simulink model "SEA_system_MPC_PID"  (R2023b)
settings: Solver=VariableStepAuto  StartTime=0.0  StopTime=10  FixedStep=0.005  RelTol=1e-3
values from neighbouring files (symbols this model uses):
  c1 = 0.6    [SEA_system.m]
  c2 = 0.6    [SEA_system.m]
  CoM1 = 0.117    [SEA_system.m]
  CoM2 = 0.045    [SEA_system.m]
  g = 9.81    [SEA_system.m]
  J1 = m1*L1^2/12 + m1*CoM1^2    (= 0.00579610927083)    [SEA_system.m]
  J2 = m2*L2^2/12 + m2*CoM2^2 + (mEE*(L2-CoM2)^2)    (= 0.00129963166667)    [SEA_system.m]
  k1 = 5.9*10^3    (= 5900)    [SEA_system.m]
  k2 = 5.9*10^3    (= 5900)    [SEA_system.m]
  L1 = 0.20075    [SEA_system.m]
  m1 = 0.340    (= 0.34)    [SEA_system.m]
  m2 = 0.140    (= 0.14)    [SEA_system.m]
  N1 = m1*CoM1^2 + J1 + m2*L1^2 + m2*CoM2^2 + J2    (= 0.0176755796875)    [SEA_system.m]
  N2 = m2*L1*CoM2    (= 0.001264725)    [SEA_system.m]
  N3 = m2*CoM2^2 + J2    (= 0.00158313166667)    [SEA_system.m]
libraries: simulink_extras x4, slpidlib x2, mpclib x1
settings Model: Creator=Master  LastModifiedBy=tpdnr
settings SolverCC: ZeroCrossAlgorithm=Adaptive
settings DebuggingCC: MaskedZcDiagnostic=none  IgnoredZcDiagnostic=none

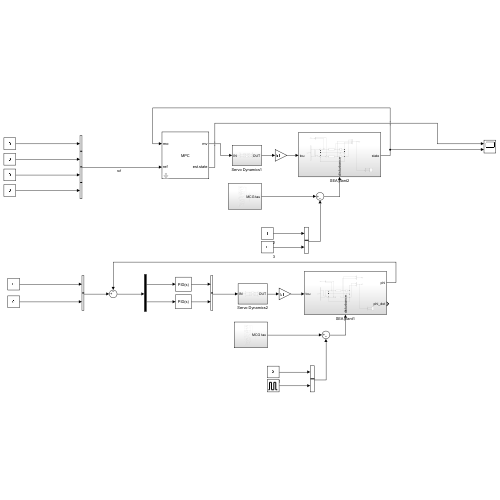
[thumbnail: Simulink's stored preview of the top-level diagram]
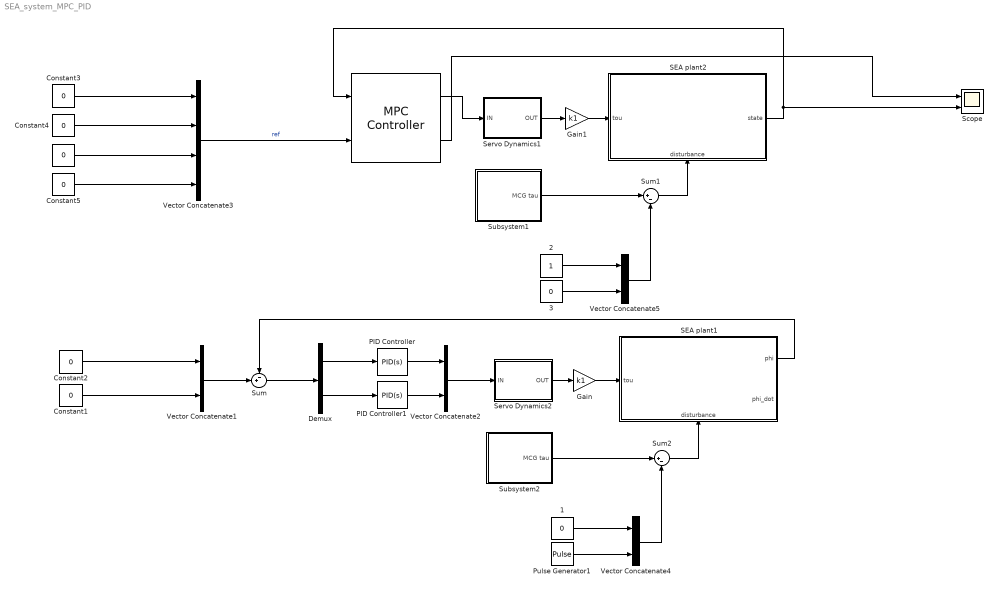
== system SEA_system_MPC_PID ==
  " " : Constant  Value=0
  "  " : mpclib/MPC Controller  SCDEnableBlockLinearizationSpecification=on  mpcobj=mpcobj  is_multiple=0  enable_value=0  return_u0=off  updateMPCinCallerWorkspace=on  md_inport=off  mv_inport=off  uref_inport=off  return_cost=off  return_mvseq=off  return_qpstatus=off  return_xseq=off  return_state=on  return_ovseq=off  state_inport=off  umin_inport=off  umax_inport=off  ymin_inport=off  ymax_inport=off  cc_inport=off  ywt_inport=off  uwt_inport=off  duwt_inport=off  rhoeps_inport=off  pm_inport=off  MaximumP=10  HorizonChoice=FixedHorizon  n_ts=0.01  n_p=10  n_mv=2  n_md=0  n_ud=0  n_mo=4  n_uo=0  BlockDataType=double  SampleTimeInherited=off  switch_inport=off
  "            1" : Constant  Value=0
  "            2" : Constant
  "            3" : Constant  Value=0
  Constant{1..5} (5 alike) : Constant  Value=0
  Demux : Demux  Outputs=2
  Gain : Gain  Gain=k1
  Gain1 : Gain  Gain=k1
  PID Controller : slpidlib/PID Controller  Controller=PID  Form=Parallel  TimeDomain=Continuous-time  UseExternalTs=off  SampleTime=-1  IntegratorMethod=Forward Euler  FilterMethod=Forward Euler  ControllerParametersSource=internal  P=5  I=1  UseKiTs=off  D=0  N=100  UseFilter=on  TunerSelectOption=Transfer Function Based (PID Tuner App)  InitialConditionSource=internal  InitialConditionForIntegrator=0  InitialConditionForFilter=0  DifferentiatorICPrevScaledInput=0  ExternalReset=none  TrackingMode=off  Kt=1  LimitOutput=off  SatLimitsSource=internal  UpperSaturationLimit=inf  LowerSaturationLimit=-inf  LinearizeAsGain=on  AntiWindupMode=none  Kb=1  LimitIntegrator=off  UpperIntegratorSaturationLimit=inf  LowerIntegratorSaturationLimit=-inf  POutMin=[]  POutMax=[]  IOutMin=[]  IOutMax=[]  DOutMin=[]  DOutMax=[]  NOutMin=[]  NOutMax=[]  SumOutMin=[]  SumOutMax=[]  SaturationOutMin=[]  SaturationOutMax=[]  PParamMin=[]  PParamMax=[]  IParamMin=[]  IParamMax=[]  DParamMin=[]  DParamMax=[]  NParamMin=[]  NParamMax=[]  KbParamMin=[]  KbParamMax=[]  KtParamMin=[]  KtParamMax=[]  KbOutMin=[]  KbOutMax=[]  KtOutMin=[]  KtOutMax=[]  IntegratorOutMin=[]  IntegratorOutMax=[]  FilterOutMin=[]  FilterOutMax=[]  SumI1OutMin=[]  SumI1OutMax=[]  SumI2OutMin=[]  SumI2OutMax=[]  SumI3OutMin=[]  SumI3OutMax=[]  SumI4OutMin=[]  SumI4OutMax=[]  SumDOutMin=[]  SumDOutMax=[]  DifferentiatorOutMin=[]  DifferentiatorOutMax=[]  FilterDiffOutCoefMin=[]  FilterDiffOutCoefMax=[]  ReciprocalOutMin=[]  ReciprocalOutMax=[]  SumDenOutMin=[]  SumDenOutMax=[]  SumNumOutMin=[]  SumNumOutMax=[]  DivideOutMin=[]  DivideOutMax=[]  UdiffTsProdOutMin=[]  UdiffTsProdOutMax=[]  NTsProdOutMin=[]  NTsProdOutMax=[]  UintegralTsProdOutMin=[]  UintegralTsProdOutMax=[]  UngainTsProdOutMin=[]  UngainTsProdOutMax=[]  ClampingZeroOutDataTypeStr=Inherit: Inherit via back propagation  ClampingZeroOutMin=[]  ClampingZeroOutMax=[]  FilterDenConstantOutDataTypeStr=Inherit: Inherit via back propagation  FilterDenConstantOutMin=[]  FilterDenConstantOutMax=[]  PCopyOutDataTypeStr=Inherit: Inherit via back propagation  PCopyOutMin=[]  PCopyOutMax=[]  NCopyOutDataTypeStr=Inherit: Inherit via back propagation  NCopyOutMin=[]  NCopyOutMax=[]  IntegratorContinuousStateAttributes=''  IntegratorStateMustResolveToSignalObject=off  IntegratorRTWStateStorageClass=Auto  FilterContinuousStateAttributes=''  FilterStateMustResolveToSignalObject=off  FilterRTWStateStorageClass=Auto  ParallelPVariant=InternalParameters  IdealPVariant=Disabled  IVariant=InternalParameters  DVariant=InternalParameters  IntegratorVariant=Continuous  SatVariant=Disabled  AWVariant=Passthrough  PCopyVariant=Disabled  TRVariant=Disabled  FdbkBlocksVariant=Forward  IdealPFdbkVariant=Disabled  SatFdbkVariant=Disabled  DerivativeFilterVariant=ContFilter  NVariant=InternalParameters  NCopyVariant=Disabled  FilterICVariant=InternalICsFilter  IntegratorICVariant=InternalICs  ExternalResetVariant=Disabled  TRSumVariant=Passthrough  SumFdbkVariant=Disabled  SumVariant=Sum_PID  TsampFilterVariant=InternalTs  TsampNgainVariant=Passthrough  TsampIntegralVariant=Disabled_SignalSpec  ExternalSaturationOutDataTypeStr=Inherit: Same as second input
  PID Controller1 : slpidlib/PID Controller  Controller=PID  Form=Parallel  TimeDomain=Continuous-time  UseExternalTs=off  SampleTime=-1  IntegratorMethod=Forward Euler  FilterMethod=Forward Euler  ControllerParametersSource=internal  P=5  I=1  UseKiTs=off  D=0  N=100  UseFilter=on  TunerSelectOption=Transfer Function Based (PID Tuner App)  InitialConditionSource=internal  InitialConditionForIntegrator=0  InitialConditionForFilter=0  DifferentiatorICPrevScaledInput=0  ExternalReset=none  TrackingMode=off  Kt=1  LimitOutput=off  SatLimitsSource=internal  UpperSaturationLimit=inf  LowerSaturationLimit=-inf  LinearizeAsGain=on  AntiWindupMode=none  Kb=1  LimitIntegrator=off  UpperIntegratorSaturationLimit=inf  LowerIntegratorSaturationLimit=-inf  POutMin=[]  POutMax=[]  IOutMin=[]  IOutMax=[]  DOutMin=[]  DOutMax=[]  NOutMin=[]  NOutMax=[]  SumOutMin=[]  SumOutMax=[]  SaturationOutMin=[]  SaturationOutMax=[]  PParamMin=[]  PParamMax=[]  IParamMin=[]  IParamMax=[]  DParamMin=[]  DParamMax=[]  NParamMin=[]  NParamMax=[]  KbParamMin=[]  KbParamMax=[]  KtParamMin=[]  KtParamMax=[]  KbOutMin=[]  KbOutMax=[]  KtOutMin=[]  KtOutMax=[]  IntegratorOutMin=[]  IntegratorOutMax=[]  FilterOutMin=[]  FilterOutMax=[]  SumI1OutMin=[]  SumI1OutMax=[]  SumI2OutMin=[]  SumI2OutMax=[]  SumI3OutMin=[]  SumI3OutMax=[]  SumI4OutMin=[]  SumI4OutMax=[]  SumDOutMin=[]  SumDOutMax=[]  DifferentiatorOutMin=[]  DifferentiatorOutMax=[]  FilterDiffOutCoefMin=[]  FilterDiffOutCoefMax=[]  ReciprocalOutMin=[]  ReciprocalOutMax=[]  SumDenOutMin=[]  SumDenOutMax=[]  SumNumOutMin=[]  SumNumOutMax=[]  DivideOutMin=[]  DivideOutMax=[]  UdiffTsProdOutMin=[]  UdiffTsProdOutMax=[]  NTsProdOutMin=[]  NTsProdOutMax=[]  UintegralTsProdOutMin=[]  UintegralTsProdOutMax=[]  UngainTsProdOutMin=[]  UngainTsProdOutMax=[]  ClampingZeroOutDataTypeStr=Inherit: Inherit via back propagation  ClampingZeroOutMin=[]  ClampingZeroOutMax=[]  FilterDenConstantOutDataTypeStr=Inherit: Inherit via back propagation  FilterDenConstantOutMin=[]  FilterDenConstantOutMax=[]  PCopyOutDataTypeStr=Inherit: Inherit via back propagation  PCopyOutMin=[]  PCopyOutMax=[]  NCopyOutDataTypeStr=Inherit: Inherit via back propagation  NCopyOutMin=[]  NCopyOutMax=[]  IntegratorContinuousStateAttributes=''  IntegratorStateMustResolveToSignalObject=off  IntegratorRTWStateStorageClass=Auto  FilterContinuousStateAttributes=''  FilterStateMustResolveToSignalObject=off  FilterRTWStateStorageClass=Auto  ParallelPVariant=InternalParameters  IdealPVariant=Disabled  IVariant=InternalParameters  DVariant=InternalParameters  IntegratorVariant=Continuous  SatVariant=Disabled  AWVariant=Passthrough  PCopyVariant=Disabled  TRVariant=Disabled  FdbkBlocksVariant=Forward  IdealPFdbkVariant=Disabled  SatFdbkVariant=Disabled  DerivativeFilterVariant=ContFilter  NVariant=InternalParameters  NCopyVariant=Disabled  FilterICVariant=InternalICsFilter  IntegratorICVariant=InternalICs  ExternalResetVariant=Disabled  TRSumVariant=Passthrough  SumFdbkVariant=Disabled  SumVariant=Sum_PID  TsampFilterVariant=InternalTs  TsampNgainVariant=Passthrough  TsampIntegralVariant=Disabled_SignalSpec  ExternalSaturationOutDataTypeStr=Inherit: Same as second input
  Pulse Generator1 : DiscretePulseGenerator  PulseType=Time based  Amplitude=0.0000000000000000000000000000000000000000001  Period=10  PulseWidth=5  PhaseDelay=3
  SEA plant1 : Subsystem
      settings: PortSchema="{\"entries\":[{\"content\":{\"sides\":[{\"content\":{\"connectorIds\":[\"In1\"]},\"type\":\"ConnectorPlacement.EquallySpacedRectSide\",\"uuid\":\"1b93464f-37dd-43a9-ab32-27cc58323ee6\"},{\"content\":{\"connectorIds\":[\"Out1\",\"Out2\"],\"side\":\"RIGHT\"},\"type\":\"ConnectorPlacement.EquallySpacedRectSide\",\"uuid\":\"bb6cc86c-e995-4dd3-b7ed-185a956ec5b1\"},{\"content\":{\"side\":\"TOP\"},\"type\":\"ConnectorPlacement.EquallySpacedRectSide\",\"uuid\":\"aadabb70-89b6-4b18-b344-efc0c5c70e88\"},{\"content\":{\"connectorIds\":[\"In2\"],\"side\":\"BOTTOM\"},\"type\":\"ConnectorPlacement.EquallySpacedRectSide\",\"uuid\":\"f54ebc4c-f8c7-49d2-9ddc-bd8b86e29db6\"}]},\"type\":\"ConnectorPlacement.EquallySpacedConnector\",\"uuid\":\"e4bf620f-c290-4875-9798-b5a7df6de3ac\"}],\"packageUris\":[\"http://schema.mathworks.com/mf0/Connector/R2020b\"],\"version\":\"1.0\"}"
  SEA plant2 : Subsystem
      settings: PortSchema="{\"entries\":[{\"content\":{\"sides\":[{\"content\":{\"connectorIds\":[\"In1\"]},\"type\":\"ConnectorPlacement.EquallySpacedRectSide\",\"uuid\":\"4f8d15b8-84da-4bfe-9413-20834dd5d7ae\"},{\"content\":{\"connectorIds\":[\"Out1\"],\"side\":\"RIGHT\"},\"type\":\"ConnectorPlacement.EquallySpacedRectSide\",\"uuid\":\"3b7a460f-373c-467c-a170-5be31d779b4c\"},{\"content\":{\"side\":\"TOP\"},\"type\":\"ConnectorPlacement.EquallySpacedRectSide\",\"uuid\":\"85d4de2f-2986-450f-b49e-1b05e10c32b4\"},{\"content\":{\"connectorIds\":[\"In2\"],\"side\":\"BOTTOM\"},\"type\":\"ConnectorPlacement.EquallySpacedRectSide\",\"uuid\":\"ce7f6b74-1213-403d-8fa7-cc43fa584a7b\"}]},\"type\":\"ConnectorPlacement.EquallySpacedConnector\",\"uuid\":\"d903d6ae-f821-4d4f-a02b-62e0c83e6cea\"}],\"packageUris\":[\"http://schema.mathworks.com/mf0/Connector/R2020b\"],\"version\":\"1.0\"}"
  Scope : Scope  NumInputPorts=2
  Servo Dynamics1 : Subsystem
  Servo Dynamics2 : Subsystem
  Subsystem1 : Subsystem
  Subsystem2 : Subsystem
  Sum : Sum  Inputs=-+|
  Sum1 : Sum  Inputs=|+-
  Sum2 : Sum  Inputs=|+-
  Vector Concatenate{1..2,4..5} (4 alike) : Concatenate
  Vector Concatenate3 : Concatenate  NumInputs=4
  wires:
  Servo Dynamics1/1(OUT) -> Gain1/1
  "  "/1 -> Servo Dynamics1/1(IN)
  Vector Concatenate3/1 -> "  "/2  "ref"
  Servo Dynamics2/1(OUT) -> Gain/1
  Constant2/1 -> Vector Concatenate1/1
  Constant1/1 -> Vector Concatenate1/2
  Vector Concatenate1/1 -> Sum/2
  SEA plant1/1(phi) -> Sum/1
  SEA plant2/1(state) -> Scope/2, "  "/1
  PID Controller/1 -> Vector Concatenate2/1
  PID Controller1/1 -> Vector Concatenate2/2
  Vector Concatenate2/1 -> Servo Dynamics2/1(IN)
  Demux/1 -> PID Controller/1
  Demux/2 -> PID Controller1/1
  Sum/1 -> Demux/1
  Constant3/1 -> Vector Concatenate3/1
  " "/1 -> Vector Concatenate3/3
  Constant4/1 -> Vector Concatenate3/2
  Constant5/1 -> Vector Concatenate3/4
  Gain/1 -> SEA plant1/1(tou)
  Gain1/1 -> SEA plant2/1(tou)
  Pulse Generator1/1 -> Vector Concatenate4/2
  "            1"/1 -> Vector Concatenate4/1
  Sum2/1 -> SEA plant1/2(disturbance)
  Vector Concatenate4/1 -> Sum2/2
  Subsystem2/1(MCG tau) -> Sum2/1
  Sum1/1 -> SEA plant2/2(disturbance)
  "            2"/1 -> Vector Concatenate5/1
  "            3"/1 -> Vector Concatenate5/2
  Subsystem1/1(MCG tau) -> Sum1/1
  Vector Concatenate5/1 -> Sum1/2
  "  "/2 -> Scope/1

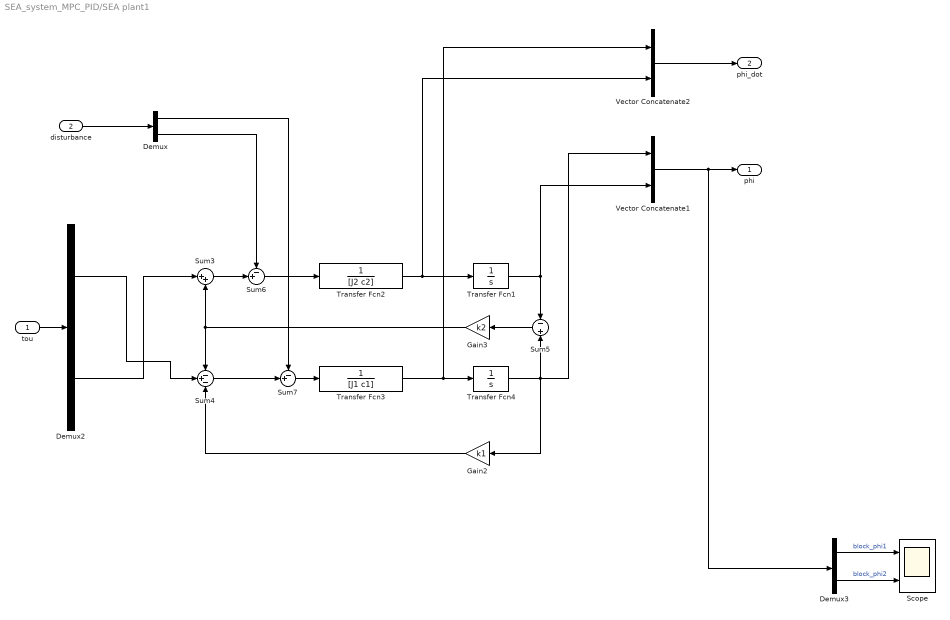
== system SEA_system_MPC_PID/SEA plant1 ==
  tou : Inport
  disturbance : Inport  Port=2
  Demux : Demux  Outputs=2
  Demux2 : Demux  Outputs=2
  Demux3 : Demux  Outputs=2
  Gain2 : Gain  Gain=k1
  Gain3 : Gain  Gain=k2
  Scope : Scope  NumInputPorts=2
  Sum3 : Sum  Inputs=|++
  Sum4 : Sum  Inputs=-+-
  Sum5 : Sum  Inputs=-|+
  Sum6 : Sum  Inputs=-+|
  Sum7 : Sum  Inputs=-+|
  Transfer Fcn1 : TransferFcn  Denominator=[1 0]
  Transfer Fcn2 : TransferFcn  Denominator=[J2 c2]
  Transfer Fcn3 : TransferFcn  Denominator=[J1 c1]
  Transfer Fcn4 : TransferFcn  Denominator=[1 0]
  Vector Concatenate1 : Concatenate
  Vector Concatenate2 : Concatenate
  phi : Outport
  phi_dot : Outport  Port=2
  wires:
  Transfer Fcn3/1 -> Vector Concatenate2/1, Transfer Fcn4/1
  Gain3/1 -> Sum3/2, Sum4/1
  Sum6/1 -> Transfer Fcn2/1
  Transfer Fcn2/1 -> Vector Concatenate2/2, Transfer Fcn1/1
  Sum5/1 -> Gain3/1
  Vector Concatenate1/1 -> Demux3/1, phi/1
  Sum7/1 -> Transfer Fcn3/1
  Gain2/1 -> Sum4/3
  Demux2/2 -> Sum3/1
  Demux2/1 -> Sum4/2
  Sum4/1 -> Sum7/2
  tou/1 -> Demux2/1
  Transfer Fcn1/1 -> Sum5/1, Vector Concatenate1/2
  Transfer Fcn4/1 -> Gain2/1, Vector Concatenate1/1, Sum5/2
  Vector Concatenate2/1 -> phi_dot/1
  Demux3/1 -> Scope/1  "block_phi1"
  Demux3/2 -> Scope/2  "block_phi2"
  Sum3/1 -> Sum6/2
  disturbance/1 -> Demux/1
  Demux/1 -> Sum7/1
  Demux/2 -> Sum6/1

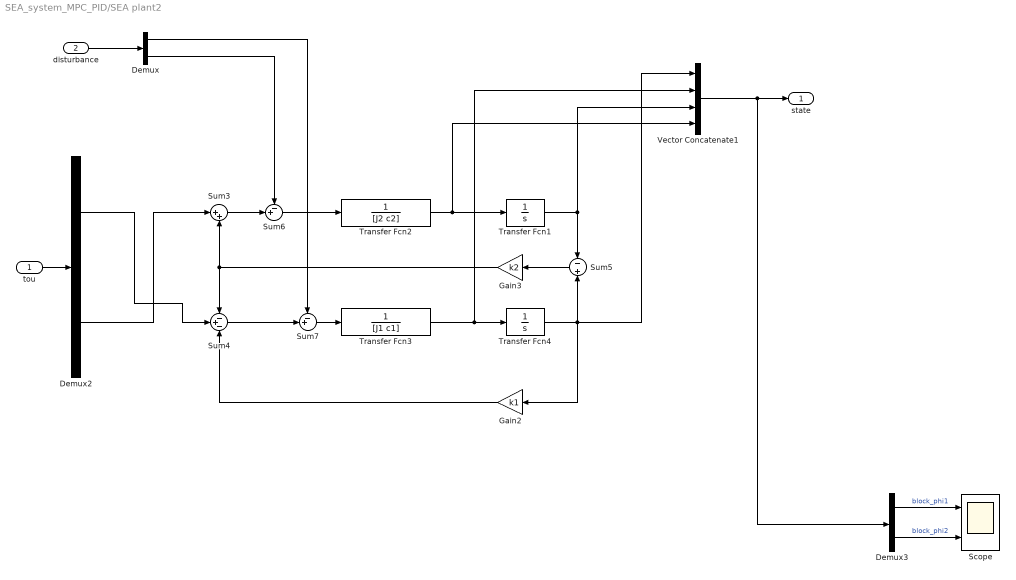
== system SEA_system_MPC_PID/SEA plant2 ==
  tou : Inport
  disturbance : Inport  Port=2
  Demux : Demux  Outputs=2
  Demux2 : Demux  Outputs=2
  Demux3 : Demux  Outputs=2
  Gain2 : Gain  Gain=k1
  Gain3 : Gain  Gain=k2
  Scope : Scope  NumInputPorts=2
  Sum3 : Sum  Inputs=|++
  Sum4 : Sum  Inputs=-+-
  Sum5 : Sum  Inputs=-|+
  Sum6 : Sum  Inputs=-+|
  Sum7 : Sum  Inputs=-+|
  Transfer Fcn1 : TransferFcn  Denominator=[1 0]
  Transfer Fcn2 : TransferFcn  Denominator=[J2 c2]
  Transfer Fcn3 : TransferFcn  Denominator=[J1 c1]
  Transfer Fcn4 : TransferFcn  Denominator=[1 0]
  Vector Concatenate1 : Concatenate  NumInputs=4
  state : Outport
  wires:
  Transfer Fcn3/1 -> Vector Concatenate1/2, Transfer Fcn4/1
  Gain3/1 -> Sum3/2, Sum4/1
  Sum6/1 -> Transfer Fcn2/1
  Transfer Fcn2/1 -> Vector Concatenate1/4, Transfer Fcn1/1
  Sum5/1 -> Gain3/1
  Vector Concatenate1/1 -> Demux3/1, state/1
  Sum7/1 -> Transfer Fcn3/1
  Gain2/1 -> Sum4/3
  Demux2/2 -> Sum3/1
  Demux2/1 -> Sum4/2
  Sum4/1 -> Sum7/2
  tou/1 -> Demux2/1
  Transfer Fcn1/1 -> Vector Concatenate1/3, Sum5/1
  Transfer Fcn4/1 -> Gain2/1, Vector Concatenate1/1, Sum5/2
  Demux3/1 -> Scope/1  "block_phi1"
  Demux3/2 -> Scope/2  "block_phi2"
  Sum3/1 -> Sum6/2
  disturbance/1 -> Demux/1
  Demux/1 -> Sum7/1
  Demux/2 -> Sum6/1

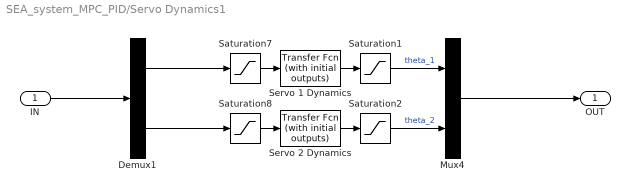
== system SEA_system_MPC_PID/Servo Dynamics1 ==
  IN : Inport
  Demux1 : Demux  Outputs=2
  Mux4 : Mux  Inputs=2
  Saturation{1..2,7..8} (4 alike) : Saturate  UpperLimit=5  LowerLimit=-5
  Servo 1 Dynamics : simulink_extras/Additional Linear/Transfer Fcn (with initial outputs)  N=[1]  D="[1/10  1]"  Y0=0  U0=0
  Servo 2 Dynamics : simulink_extras/Additional Linear/Transfer Fcn (with initial outputs)  N=[1]  D="[1/10  1]"  Y0=0  U0=0
  OUT : Outport
  wires:
  Saturation2/1 -> Mux4/2  "theta_2"
  Saturation1/1 -> Mux4/1  "theta_1"
  Saturation8/1 -> Servo 2 Dynamics/1
  Demux1/1 -> Saturation7/1
  Demux1/2 -> Saturation8/1
  Saturation7/1 -> Servo 1 Dynamics/1
  Servo 2 Dynamics/1 -> Saturation2/1
  Servo 1 Dynamics/1 -> Saturation1/1
  IN/1 -> Demux1/1
  Mux4/1 -> OUT/1

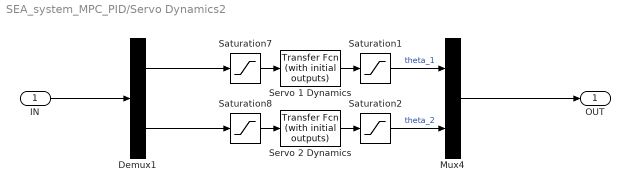
== system SEA_system_MPC_PID/Servo Dynamics2 ==
  IN : Inport
  Demux1 : Demux  Outputs=2
  Mux4 : Mux  Inputs=2
  Saturation{1..2,7..8} (4 alike) : Saturate  UpperLimit=5  LowerLimit=-5
  Servo 1 Dynamics : simulink_extras/Additional Linear/Transfer Fcn (with initial outputs)  N=[1]  D="[1/10  1]"  Y0=0  U0=0
  Servo 2 Dynamics : simulink_extras/Additional Linear/Transfer Fcn (with initial outputs)  N=[1]  D="[1/10  1]"  Y0=0  U0=0
  OUT : Outport
  wires:
  Saturation2/1 -> Mux4/2  "theta_2"
  Saturation1/1 -> Mux4/1  "theta_1"
  Saturation8/1 -> Servo 2 Dynamics/1
  Demux1/1 -> Saturation7/1
  Demux1/2 -> Saturation8/1
  Saturation7/1 -> Servo 1 Dynamics/1
  Servo 2 Dynamics/1 -> Saturation2/1
  Servo 1 Dynamics/1 -> Saturation1/1
  IN/1 -> Demux1/1
  Mux4/1 -> OUT/1

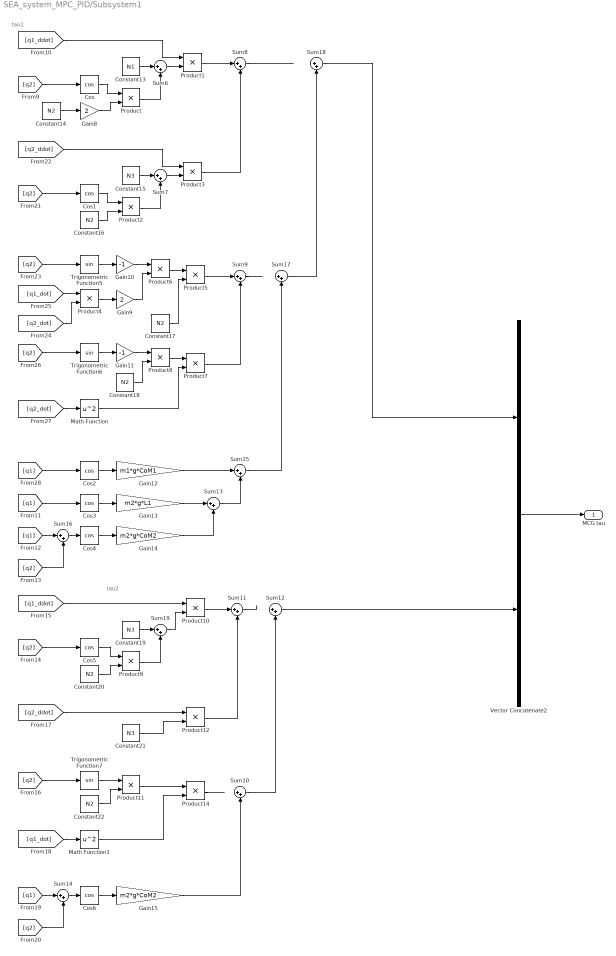
== system SEA_system_MPC_PID/Subsystem1 ==
  note: tau2
  note: tau1
  Constant13 : Constant  Value=N1
  Constant{14,16..18,20,22} (6 alike) : Constant  Value=N2
  Constant15 : Constant  Value=N3
  Constant19 : Constant  Value=N3
  Constant21 : Constant  Value=N3
  Cos{,1..6} (7 alike) : Trigonometry  Operator=cos
  Gain10 : Gain  Gain=-1
  Gain11 : Gain  Gain=-1
  Gain12 : Gain  Gain=m1*g*CoM1
  Gain13 : Gain  Gain=m2*g*L1
  Gain14 : Gain  Gain=m2*g*CoM2
  Gain15 : Gain  Gain=m2*g*CoM2
  Gain8 : Gain  Gain=2
  Gain9 : Gain  Gain=2
  Math Function : Math  Operator=square
  Math Function1 : Math  Operator=square
  Product{,1..12,14} (14 alike) : Product
  Sum{6..19} (14 alike) : Sum  Inputs=|++
  Trigonometric Function5 : Trigonometry
  Trigonometric Function6 : Trigonometry
  Trigonometric Function7 : Trigonometry
  Vector Concatenate2 : Concatenate
  MCG tau : Outport
  wires:
  Cos5/1 -> Product9/1
  Constant21/1 -> Product12/2
  Product10/1 -> Sum11/1
  [q1_ddot] -> Product10/1
  Sum11/1 -> ?
  Product12/1 -> Sum11/2
  [q1] -> Sum14/1
  Sum14/1 -> Cos6/1
  Sum10/1 -> Sum12/2
  Product9/1 -> Sum19/2
  Cos6/1 -> Gain15/1
  [q2] -> Sum14/2
  Gain15/1 -> Sum10/2
  [q1_dot] -> Math Function1/1
  Math Function1/1 -> Product14/2
  Constant20/1 -> Product9/2
  [q2_ddot] -> Product12/1
  [q2] -> Cos5/1
  Product11/1 -> Product14/1
  [q2] -> Trigonometric Function7/1
  Trigonometric Function7/1 -> Product11/1
  Constant22/1 -> Product11/2
  Constant19/1 -> Sum19/1
  Product14/1 -> ?
  Sum19/1 -> Product10/2
  Constant17/1 -> Product5/2
  Constant14/1 -> Gain8/1
  Cos4/1 -> Gain14/1
  Product7/1 -> Sum9/2
  Sum17/1 -> Sum18/2
  [q2_dot] -> Math Function/1
  [q1] -> Cos3/1
  Cos/1 -> Product/1
  Product4/1 -> Gain9/1
  Product8/1 -> Product7/1
  [q1_dot] -> Product4/1
  Gain10/1 -> Product6/1
  Constant15/1 -> Sum7/1
  Sum8/1 -> ?
  Math Function/1 -> Product7/2
  Cos3/1 -> Gain13/1
  Gain12/1 -> Sum15/1
  Sum16/1 -> Cos4/1
  [q1] -> Cos2/1
  Product1/1 -> Sum8/1
  [q2] -> Sum16/2
  [q1] -> Sum16/1
  [q2] -> Trigonometric Function6/1
  Product5/1 -> Sum9/1
  Sum13/1 -> Sum15/2
  [q2_dot] -> Product4/2
  Trigonometric Function5/1 -> Gain10/1
  Product/1 -> Sum6/2
  Gain11/1 -> Product8/1
  Sum6/1 -> Product1/2
  Product6/1 -> Product5/1
  Sum9/1 -> ?
  Gain9/1 -> Product6/2
  Trigonometric Function6/1 -> Gain11/1
  Product3/1 -> Sum8/2
  Gain8/1 -> Product/2
  Constant16/1 -> Product2/2
  Constant18/1 -> Product8/2
  Cos1/1 -> Product2/1
  Cos2/1 -> Gain12/1
  Constant13/1 -> Sum6/1
  [q2] -> Cos1/1
  Sum7/1 -> Product3/2
  Gain14/1 -> Sum13/2
  Product2/1 -> Sum7/2
  [q2] -> Trigonometric Function5/1
  [q2_ddot] -> Product3/1
  Sum15/1 -> Sum17/2
  [q2] -> Cos/1
  Gain13/1 -> Sum13/1
  [q1_ddot] -> Product1/1
  Sum18/1 -> Vector Concatenate2/1
  Sum12/1 -> Vector Concatenate2/2
  Vector Concatenate2/1 -> MCG tau/1

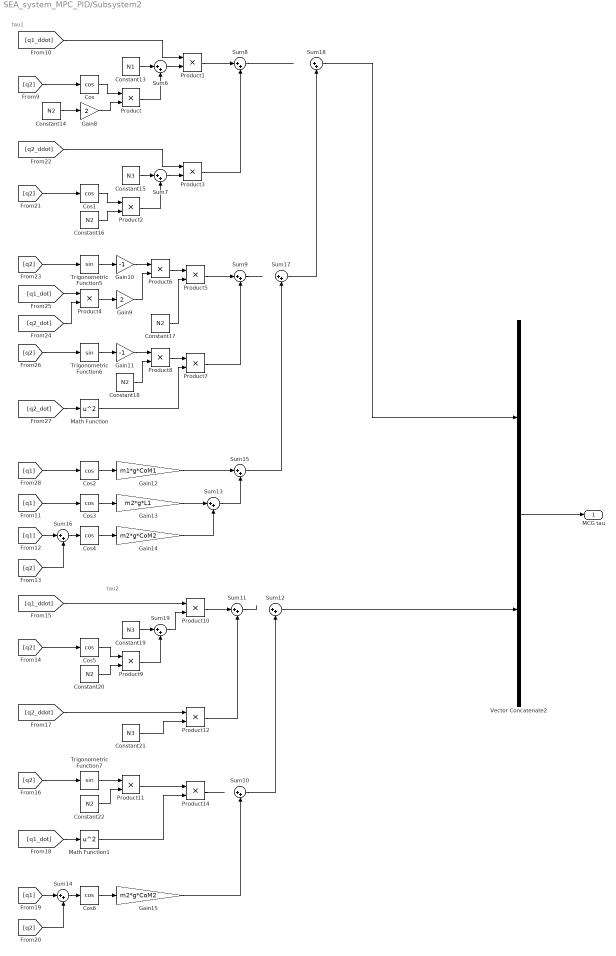
== system SEA_system_MPC_PID/Subsystem2 ==
  note: tau2
  note: tau1
  Constant13 : Constant  Value=N1
  Constant{14,16..18,20,22} (6 alike) : Constant  Value=N2
  Constant15 : Constant  Value=N3
  Constant19 : Constant  Value=N3
  Constant21 : Constant  Value=N3
  Cos{,1..6} (7 alike) : Trigonometry  Operator=cos
  Gain10 : Gain  Gain=-1
  Gain11 : Gain  Gain=-1
  Gain12 : Gain  Gain=m1*g*CoM1
  Gain13 : Gain  Gain=m2*g*L1
  Gain14 : Gain  Gain=m2*g*CoM2
  Gain15 : Gain  Gain=m2*g*CoM2
  Gain8 : Gain  Gain=2
  Gain9 : Gain  Gain=2
  Math Function : Math  Operator=square
  Math Function1 : Math  Operator=square
  Product{,1..12,14} (14 alike) : Product
  Sum{6..19} (14 alike) : Sum  Inputs=|++
  Trigonometric Function5 : Trigonometry
  Trigonometric Function6 : Trigonometry
  Trigonometric Function7 : Trigonometry
  Vector Concatenate2 : Concatenate
  MCG tau : Outport
  wires:
  Cos5/1 -> Product9/1
  Constant21/1 -> Product12/2
  Product10/1 -> Sum11/1
  [q1_ddot] -> Product10/1
  Sum11/1 -> ?
  Product12/1 -> Sum11/2
  [q1] -> Sum14/1
  Sum14/1 -> Cos6/1
  Sum10/1 -> Sum12/2
  Product9/1 -> Sum19/2
  Cos6/1 -> Gain15/1
  [q2] -> Sum14/2
  Gain15/1 -> Sum10/2
  [q1_dot] -> Math Function1/1
  Math Function1/1 -> Product14/2
  Constant20/1 -> Product9/2
  [q2_ddot] -> Product12/1
  [q2] -> Cos5/1
  Product11/1 -> Product14/1
  [q2] -> Trigonometric Function7/1
  Trigonometric Function7/1 -> Product11/1
  Constant22/1 -> Product11/2
  Constant19/1 -> Sum19/1
  Product14/1 -> ?
  Sum19/1 -> Product10/2
  Constant17/1 -> Product5/2
  Constant14/1 -> Gain8/1
  Cos4/1 -> Gain14/1
  Product7/1 -> Sum9/2
  Sum17/1 -> Sum18/2
  [q2_dot] -> Math Function/1
  [q1] -> Cos3/1
  Cos/1 -> Product/1
  Product4/1 -> Gain9/1
  Product8/1 -> Product7/1
  [q1_dot] -> Product4/1
  Gain10/1 -> Product6/1
  Constant15/1 -> Sum7/1
  Sum8/1 -> ?
  Math Function/1 -> Product7/2
  Cos3/1 -> Gain13/1
  Gain12/1 -> Sum15/1
  Sum16/1 -> Cos4/1
  [q1] -> Cos2/1
  Product1/1 -> Sum8/1
  [q2] -> Sum16/2
  [q1] -> Sum16/1
  [q2] -> Trigonometric Function6/1
  Product5/1 -> Sum9/1
  Sum13/1 -> Sum15/2
  [q2_dot] -> Product4/2
  Trigonometric Function5/1 -> Gain10/1
  Product/1 -> Sum6/2
  Gain11/1 -> Product8/1
  Sum6/1 -> Product1/2
  Product6/1 -> Product5/1
  Sum9/1 -> ?
  Gain9/1 -> Product6/2
  Trigonometric Function6/1 -> Gain11/1
  Product3/1 -> Sum8/2
  Gain8/1 -> Product/2
  Constant16/1 -> Product2/2
  Constant18/1 -> Product8/2
  Cos1/1 -> Product2/1
  Cos2/1 -> Gain12/1
  Constant13/1 -> Sum6/1
  [q2] -> Cos1/1
  Sum7/1 -> Product3/2
  Gain14/1 -> Sum13/2
  Product2/1 -> Sum7/2
  [q2] -> Trigonometric Function5/1
  [q2_ddot] -> Product3/1
  Sum15/1 -> Sum17/2
  [q2] -> Cos/1
  Gain13/1 -> Sum13/1
  [q1_ddot] -> Product1/1
  Sum18/1 -> Vector Concatenate2/1
  Sum12/1 -> Vector Concatenate2/2
  Vector Concatenate2/1 -> MCG tau/1
